simulink model "rMotorTemperatureDerate"  (R2024b)
settings: configuration reference "STM32H7_Config" (kept outside this file)
settings Model: DataDictionary=Master_Dictionary.sldd  EnableAccessToBaseWorkspace=off  Creator=torni  LastModifiedBy=William
settings ConfigSetRef: SourceName=STM32H7_Config

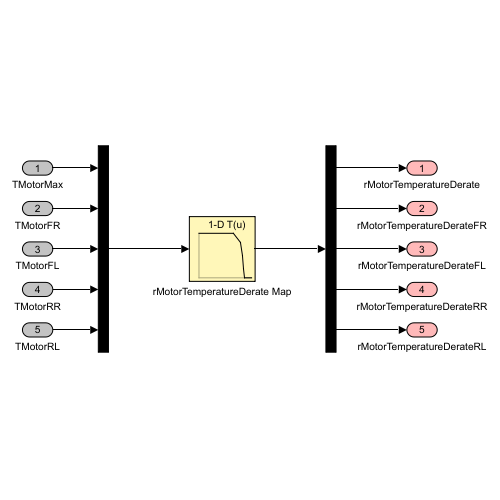
[thumbnail: Simulink's stored preview of the top-level diagram]
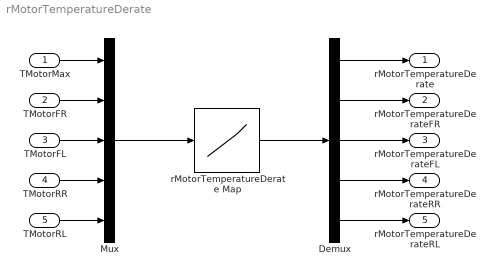
== system rMotorTemperatureDerate ==
  "TMotorMax " : Inport  OutDataTypeStr=double
  TMotorFR : Inport  Port=2  OutDataTypeStr=double
  TMotorFL : Inport  Port=3  OutDataTypeStr=double
  TMotorRR : Inport  Port=4  OutDataTypeStr=double
  TMotorRL : Inport  Port=5  OutDataTypeStr=double
  Demux : Demux  Outputs=5
  Mux : Mux  Inputs=5
  rMotorTemperatureDerate Map : Lookup_n-D  NumberOfTableDimensions=1  BreakpointsForDimension1=[0,100,120,126,128,130,150]  Table=[1,1,0.8,0.5,0.2,0,0]  InternalRulePriority=Speed  RndMeth=Simplest
  rMotorTemperatureDerate : Outport  OutDataTypeStr=double  VectorParamsAs1DForOutWhenUnconnected=off
  rMotorTemperatureDerateFR : Outport  Port=2  OutDataTypeStr=double  VectorParamsAs1DForOutWhenUnconnected=off
  rMotorTemperatureDerateFL : Outport  Port=3  OutDataTypeStr=double  VectorParamsAs1DForOutWhenUnconnected=off
  rMotorTemperatureDerateRR : Outport  Port=4  OutDataTypeStr=double  VectorParamsAs1DForOutWhenUnconnected=off
  rMotorTemperatureDerateRL : Outport  Port=5  OutDataTypeStr=double  VectorParamsAs1DForOutWhenUnconnected=off
  wires:
  TMotorFL/1 -> Mux/3
  TMotorFR/1 -> Mux/2
  "TMotorMax "/1 -> Mux/1
  Demux/1 -> rMotorTemperatureDerate/1
  Demux/5 -> rMotorTemperatureDerateRL/1
  Mux/1 -> rMotorTemperatureDerate Map/1
  Demux/3 -> rMotorTemperatureDerateFL/1
  Demux/4 -> rMotorTemperatureDerateRR/1
  TMotorRR/1 -> Mux/4
  rMotorTemperatureDerate Map/1 -> Demux/1
  Demux/2 -> rMotorTemperatureDerateFR/1
  TMotorRL/1 -> Mux/5
